simulink model "Rossler_model"  (R2023a)
settings: Solver=FixedStepAuto  StartTime=0.0  StopTime=StopTime  FixedStep=10e-4  RelTol=1e-3
PreLoadFcn:
  | run('Rossler_model_params.m');
values from neighbouring files (symbols this model uses):
  a = 0.2    [Rossler_model_params.m]    (also in Rossler_params.m)
  b = 0.2    [Rossler_model_params.m]    (also in Rossler_params.m)
  c = 5.7    [Rossler_model_params.m]    (also in Rossler_params.m)
  NoiseBit = 1    [Rossler_model_params.m]
libraries: simulink x3
settings Model: Creator=User  LastModifiedBy=jakub

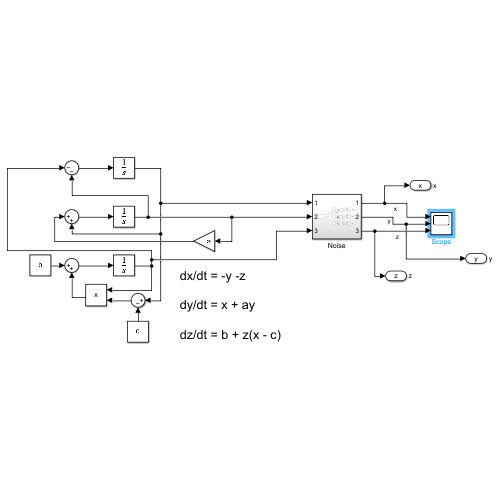
[thumbnail: Simulink's stored preview of the top-level diagram]
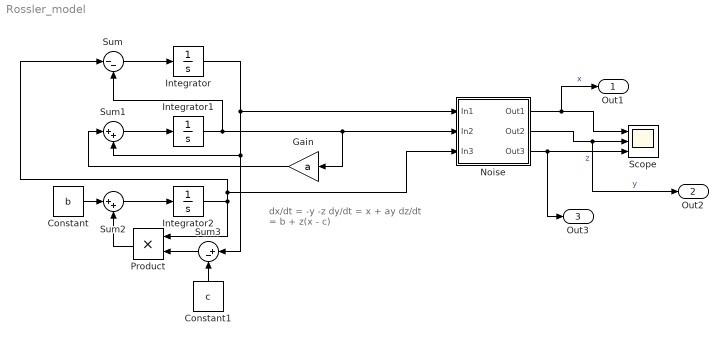
== system Rossler_model ==
  note: dx/dt = -y -z
      |
      | dy/dt = x + ay
      |
      | dz/dt = b + z(x - c)
  Constant : Constant  Value=b
  Constant1 : Constant  Value=c
  Gain : Gain  Gain=a
  Integrator : Integrator
  Integrator1 : Integrator
  Integrator2 : Integrator
  Noise : Subsystem
  Product : Product
  Scope : Scope  NumInputPorts=3
  Sum : Sum  Inputs=|--
  Sum1 : Sum  Inputs=|++
  Sum2 : Sum  Inputs=|++
  Sum3 : Sum  Inputs=|+-
  Out1 : Outport  SignalName=x
  Out2 : Outport  Port=2  SignalName=y
  Out3 : Outport  Port=3  SignalName=z
  wires:
  Sum/1 -> Integrator/1
  Integrator2/1 -> Product/1, Noise/3(In3), Sum/1
  Integrator1/1 -> Gain/1, Noise/2(In2), Sum/2
  Sum1/1 -> Integrator1/1
  Integrator/1 -> Sum1/2, Sum3/1, Noise/1(In1)
  Sum2/1 -> Integrator2/1
  Constant1/1 -> Sum3/2
  Sum3/1 -> Product/2
  Product/1 -> Sum2/2
  Constant/1 -> Sum2/1
  Gain/1 -> Sum1/1
  Noise/1(Out1) -> Out1/1, Scope/1  "x"
  Noise/2(Out2) -> Out2/1, Scope/2  "y"
  Noise/3(Out3) -> Out3/1, Scope/3  "z"

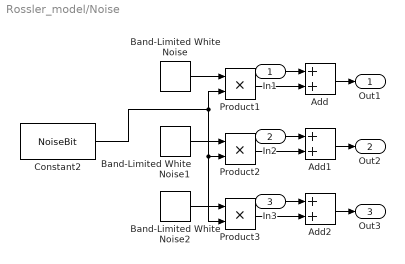
== system Rossler_model/Noise ==
  In1 : Inport
  In2 : Inport  Port=2
  In3 : Inport  Port=3
  Add : Sum
  Add1 : Sum
  Add2 : Sum
  Band-Limited White Noise : simulink/Sources/Band-Limited White Noise  Cov=NoiseLevel  Ts=0.02  seed=[23341]
  Band-Limited White Noise1 : simulink/Sources/Band-Limited White Noise  Cov=NoiseLevel  Ts=0.02  seed=[23341]
  Band-Limited White Noise2 : simulink/Sources/Band-Limited White Noise  Cov=NoiseLevel  Ts=0.02  seed=[23341]
  Constant2 : Constant  Value=NoiseBit
  Product1 : Product
  Product2 : Product
  Product3 : Product
  Out1 : Outport
  Out2 : Outport  Port=2
  Out3 : Outport  Port=3
  wires:
  In2/1 -> Add1/1
  Constant2/1 -> Product2/2, Product3/2, Product1/2
  Add/1 -> Out1/1
  Product2/1 -> Add1/2
  Band-Limited White Noise2/1 -> Product3/1
  Product1/1 -> Add/2
  Band-Limited White Noise1/1 -> Product2/1
  Product3/1 -> Add2/2
  Band-Limited White Noise/1 -> Product1/1
  Add2/1 -> Out3/1
  In3/1 -> Add2/1
  In1/1 -> Add/1
  Add1/1 -> Out2/1
